simulink model "FindPlacetoGo"  (R2020b)
settings: Solver=VariableStepAuto  StartTime=0.0  StopTime=10.0  RelTol=1e-3
libraries: aerolibguid x1
settings Model: Creator=macra  LastModifiedBy=macra

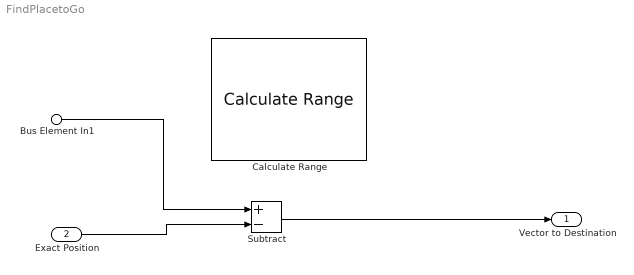
== system FindPlacetoGo ==
  Bus Element In1 : Inport  PortName=Map Data
  Exact Position : Inport  Port=2
  Calculate Range : aerolibguid/Calculate Range
      settings: SourceProductBaseCode=AE
  Subtract : Sum  Inputs=+-
  Vector to Destination : Outport
  wires:
  Subtract/1 -> Vector to Destination/1
  Bus Element In1/1 -> Subtract/1
  Exact Position/1 -> Subtract/2
